simulink model "plant"  (R2023a)
settings: Solver=FixedStepAuto  StartTime=0.0  StopTime=SIMTIME  FixedStep=SIMSTEP  RelTol=1e-3
undefined symbols (not defined in the file): A, B, bias, Bv, C, ref, wave_ampl, wave_length, x0
settings Model: Creator=X20  LastModifiedBy=X20
settings DataIOCC: ReturnWorkspaceOutputs=off

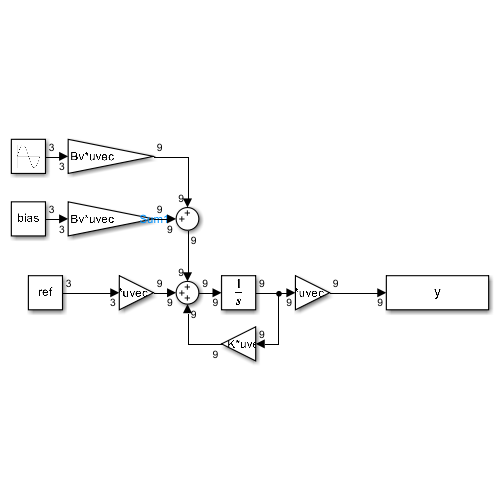
[thumbnail: Simulink's stored preview of the top-level diagram]
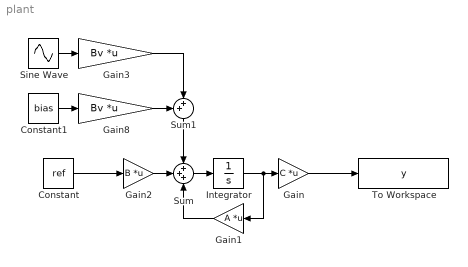
== system plant ==
  Constant : Constant  Value=ref
  Constant1 : Constant  Value=bias
  Gain : Gain  Gain=C  Multiplication=Matrix(K*u) (u vector)
  Gain1 : Gain  Gain=A  Multiplication=Matrix(K*u) (u vector)
  Gain2 : Gain  Gain=B  Multiplication=Matrix(K*u) (u vector)
  Gain3 : Gain  Gain=Bv  Multiplication=Matrix(K*u) (u vector)
  Gain8 : Gain  Gain=Bv  Multiplication=Matrix(K*u) (u vector)
  Integrator : Integrator  InitialCondition=x0
  Sine Wave : Sin  Amplitude=wave_ampl  Frequency=1./wave_length  SampleTime=0
  Sum : Sum  Inputs=+++
  Sum1 : Sum  Inputs=++|
  To Workspace : ToWorkspace  VariableName=y  SaveFormat=Timeseries  SampleTime=-1
  wires:
  Sum/1 -> Integrator/1
  Gain1/1 -> Sum/3
  Constant1/1 -> Gain8/1
  Constant/1 -> Gain2/1
  Integrator/1 -> Gain/1, Gain1/1
  Gain/1 -> To Workspace/1
  Gain2/1 -> Sum/2
  Sine Wave/1 -> Gain3/1
  Gain8/1 -> Sum1/1
  Sum1/1 -> Sum/1
  Gain3/1 -> Sum1/2
